simulink model "Seminar3_Part2_simple"  (R2023a)
settings: Solver=VariableStepAuto  StartTime=0.0  StopTime=0.2  RelTol=1e-3
libraries: spsFourierLib x12, spsIGBTDiodeLib x6, spsVoltageMeasurementLib x6, spsCurrentMeasurementLib x3, spsDCVoltageSourceLib x2, spsThreePhaseSeriesRLCBranchLib x1, sps_lib x1
settings Model: Creator=DELL  LastModifiedBy=11094
settings DataIOCC: ReturnWorkspaceOutputs=off
settings OptimizationCC: ReuseModelBlockBuffer=off

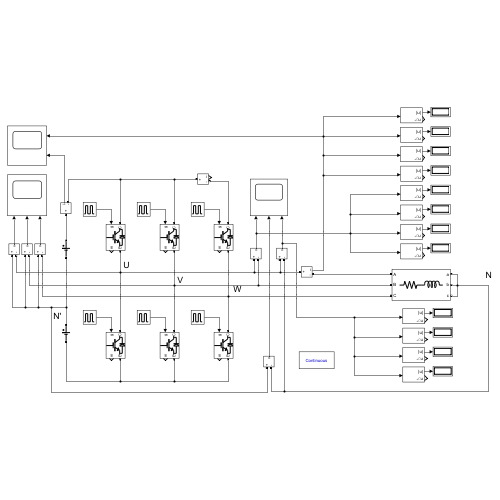
[thumbnail: Simulink's stored preview of the top-level diagram]
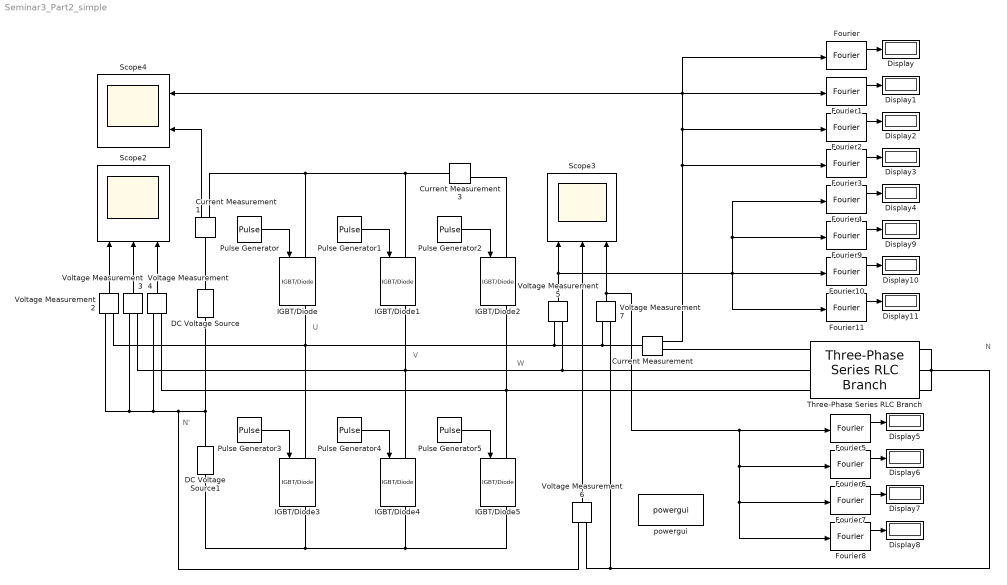
== system Seminar3_Part2_simple ==
  note: N'
  note: U
  note: V
  note: W
  note: N
  Current Measurement : spsCurrentMeasurementLib/Current Measurement  PhasorSimulation=off  OutputType=Complex  PSBequivalent=0
  Current Measurement1 : spsCurrentMeasurementLib/Current Measurement  PhasorSimulation=off  OutputType=Complex  PSBequivalent=0
  Current Measurement3 : spsCurrentMeasurementLib/Current Measurement  PhasorSimulation=off  OutputType=Complex  PSBequivalent=0
  DC Voltage Source : spsDCVoltageSourceLib/DC Voltage Source  Amplitude=100  Measurements=None
  DC Voltage Source1 : spsDCVoltageSourceLib/DC Voltage Source  Amplitude=100  Measurements=None
  Display{,1..11} (12 alike) : Display
  Fourier : spsFourierLib/Fourier  Freq=50  n=5  InInit=[0, 0]  Ts=0
  Fourier1 : spsFourierLib/Fourier  Freq=50  n=7  InInit=[0, 0]  Ts=0
  Fourier10 : spsFourierLib/Fourier  Freq=50  n=11  InInit=[0, 0]  Ts=0
  Fourier11 : spsFourierLib/Fourier  Freq=50  n=13  InInit=[0, 0]  Ts=0
  Fourier2 : spsFourierLib/Fourier  Freq=50  n=11  InInit=[0, 0]  Ts=0
  Fourier3 : spsFourierLib/Fourier  Freq=50  n=13  InInit=[0, 0]  Ts=0
  Fourier4 : spsFourierLib/Fourier  Freq=50  n=5  InInit=[0, 0]  Ts=0
  Fourier5 : spsFourierLib/Fourier  Freq=50  n=5  InInit=[0, 0]  Ts=0
  Fourier6 : spsFourierLib/Fourier  Freq=50  n=7  InInit=[0, 0]  Ts=0
  Fourier7 : spsFourierLib/Fourier  Freq=50  n=11  InInit=[0, 0]  Ts=0
  Fourier8 : spsFourierLib/Fourier  Freq=50  n=13  InInit=[0, 0]  Ts=0
  Fourier9 : spsFourierLib/Fourier  Freq=50  n=7  InInit=[0, 0]  Ts=0
  IGBT/Diode{,1..5} (6 alike) : spsIGBTDiodeLib/IGBT//Diode  Ron=1e-3  Rs=1e5  Cs=inf  Measurements=on
  Pulse Generator : DiscretePulseGenerator  PulseType=Time based  Period=0.02  PulseWidth=50
  Pulse Generator1 : DiscretePulseGenerator  PulseType=Time based  Period=0.02  PulseWidth=50  PhaseDelay=0.02/3
  Pulse Generator2 : DiscretePulseGenerator  PulseType=Time based  Period=0.02  PulseWidth=50  PhaseDelay=0.02/6+0.01
  Pulse Generator3 : DiscretePulseGenerator  PulseType=Time based  Period=0.02  PulseWidth=50  PhaseDelay=0.01
  Pulse Generator4 : DiscretePulseGenerator  PulseType=Time based  Period=0.02  PulseWidth=50  PhaseDelay=0.1/6
  Pulse Generator5 : DiscretePulseGenerator  PulseType=Time based  Period=0.02  PulseWidth=50  PhaseDelay=0.02/6
  Scope2 : Scope  NumInputPorts=3
  Scope3 : Scope  NumInputPorts=3
  Scope4 : Scope  NumInputPorts=2
  Three-Phase Series RLC Branch : spsThreePhaseSeriesRLCBranchLib/Three-Phase Series RLC Branch  LConnTagsString=A|B|C  RConnTagsString=A|B|C  BranchType=RL  Resistance=10  Inductance=0.001  Capacitance=1e-6  Measurements=None
  Voltage Measurement{2..7} (6 alike) : spsVoltageMeasurementLib/Voltage Measurement  PhasorSimulation=off  OutputType=Complex  PSBequivalent=0
  powergui : sps_lib/powergui  Priority=1  SimulationMode=Continuous  SampleTime=50e-6  frequency=60  Iterations=50  frequencyindice=0  Pbase=100e6  ErrMax=1e-4  UnitsV=kV  UnitsW=MW  buscounter=0  FunctionMessages=off  echomessages=off  EnableUseOfTLC=off  CurrentSourceSwitches=off  DisableSnubberDevices=off  DisableRonSwitches=off  DisableVfSwitches=off  DisplayEquations=off  AutomaticDiscreteSolvers=off  SolverType=Tustin/Backward Euler (TBE)  Interpol=off  ExternalGateDelay=off  methode=off  Ts=100  x0status=blocks  SPID=on  SwTol=0  HookPort=off  NonlinearTolerance=1e-4  nMaxIteration=100  ContinueOnMaxIteration=off  RestoreLinks=warning  ResistiveCurrentMeasurement=off  Frange=[0:2:500]  Ylog=off  Xlog=on  ShowGrid=off  save=off  variable=ZData  structure=0  ZoomFFT=off  StartTime=0.0  cycles=1  DisplayStyle=1  fundamental=60  FreqAxis=off  MaxFrequency=1000  frequencyindicesteady=1  RmsSteady=1  display=off
  wires:
  Pulse Generator/1 -> IGBT/Diode/1
  Pulse Generator1/1 -> IGBT/Diode1/1
  Pulse Generator4/1 -> IGBT/Diode4/1
  Pulse Generator5/1 -> IGBT/Diode5/1
  Pulse Generator2/1 -> IGBT/Diode2/1
  Pulse Generator3/1 -> IGBT/Diode3/1
  Current Measurement/1 -> Fourier/1, Fourier1/1, Scope4/1, Fourier2/1, Fourier3/1
  Fourier/1 -> Display/1
  Fourier1/1 -> Display1/1
  Fourier2/1 -> Display2/1
  Fourier3/1 -> Display3/1
  Fourier7/1 -> Display7/1
  Fourier8/1 -> Display8/1
  Fourier6/1 -> Display6/1
  Fourier11/1 -> Display11/1
  Fourier9/1 -> Display9/1
  Fourier10/1 -> Display10/1
  Fourier5/1 -> Display5/1
  Fourier4/1 -> Display4/1
  Voltage Measurement2/1 -> Scope2/1
  Voltage Measurement3/1 -> Scope2/2
  Voltage Measurement4/1 -> Scope2/3
  Voltage Measurement6/1 -> Scope3/2
  Voltage Measurement7/1 -> Scope3/3, Fourier8/1, Fourier7/1, Fourier6/1, Fourier5/1
  Current Measurement1/1 -> Scope4/2
  Voltage Measurement5/1 -> Scope3/1, Fourier9/1, Fourier4/1, Fourier11/1, Fourier10/1
  connections:
  IGBT/Diode5/RConn1 -- IGBT/Diode4/RConn1 -- DC Voltage Source1/LConn1 -- IGBT/Diode3/RConn1
  Three-Phase Series RLC Branch/RConn1 -- Voltage Measurement7/LConn2 -- Voltage Measurement6/LConn2 -- Three-Phase Series RLC Branch/RConn3 -- Three-Phase Series RLC Branch/RConn2
  IGBT/Diode4/LConn1 -- Three-Phase Series RLC Branch/LConn2 -- Voltage Measurement5/LConn2 -- Voltage Measurement3/LConn2 -- IGBT/Diode1/RConn1
  Three-Phase Series RLC Branch/LConn3 -- Voltage Measurement4/LConn2 -- IGBT/Diode5/LConn1 -- IGBT/Diode2/RConn1
  Current Measurement3/LConn1 -- Current Measurement1/RConn1 -- IGBT/Diode/LConn1 -- IGBT/Diode1/LConn1
  Current Measurement/RConn1 -- Three-Phase Series RLC Branch/LConn1
  Current Measurement/LConn1 -- Voltage Measurement7/LConn1 -- Voltage Measurement5/LConn1 -- Voltage Measurement2/LConn2 -- IGBT/Diode3/LConn1 -- IGBT/Diode/RConn1
  Current Measurement3/RConn1 -- IGBT/Diode2/LConn1
  DC Voltage Source1/RConn1 -- Voltage Measurement6/LConn1 -- Voltage Measurement2/LConn1 -- Voltage Measurement3/LConn1 -- Voltage Measurement4/LConn1 -- DC Voltage Source/LConn1
  DC Voltage Source/RConn1 -- Current Measurement1/LConn1
